simulink model "abl_M4_rigidPPC"  (R2023b)
settings: Solver=ode45  StartTime=0.0  StopTime=80  MaxStep=1e-3  RelTol=5e-5
model workspace (MAT data in the model file):
  gpsid1 : Simulink.Signal (value not decoded)
  gpsid2 : Simulink.Signal (value not decoded)
  gpsid3 : Simulink.Signal (value not decoded)
  kkk1 : Simulink.Signal (value not decoded)
  kkk2 : Simulink.Signal (value not decoded)
  kkk3 : Simulink.Signal (value not decoded)
  psid = 0.5
undefined symbols (not defined in the file): A_raw1, A_raw2, beta1, beta2, p00, p_d_10, p_d_20, p_d_30, p_d_40, p_d_50, p_d_60, p_hat_p10, p_hat_p20, p_hat_p30, p_hat_p40, p_hat_p50, p_hat_p60, p_hat_v10, p_hat_v20, p_hat_v30, p_hat_v40, p_hat_v50, p_hat_v60, p_off_set1, p_off_set2, v00
(part 3 of 4)

== matlab function abl_M4_rigidPPC/Subsystem12/Controler1 ==
  settings: updateMethod=DISCRETE
  data: t input; psi_d input; dpsid input; ddpsid input; psi_e input; rho_e input; tau_sat_rho output; tau_sat_psi output; alpha_psi output; alpha_rho output; B_psi output; B_rho output; z_rho output; desire input; u input; v input; r input; mu_rho_hat input; mu_psi_hat input; kappa_rho input; kappa_psi input; dot_mu_rho_hat output; dot_mu_psi_hat output; d_kappa_rho output; d_kappa_psi output; d_chi_rho_1 output; d_chi_rho_2 output; d_chi_psi_1 output; d_chi_psi_2 output; chi_rho_1 input; chi_rho_2 input; chi_psi_1 input; chi_psi_2 input; S_rho input; S_psi input; d_S_rho output; d_S_psi output
% function [tau_u,tau_r,alpha_psi,alpha_rho,dot_mu_rho_hat,dot_mu_psi_hat,sigma_rho,sigma_psi,z_rho,z_psi,term1 ,dpsie] = controller(t,psi_d,dpsid,ddpsid,psi_e, rho_e,desire,u, v, r,mu_rho_hat,mu_psi_hat)
% dxd = desire(2);ddxd = desire(3);dyd = desire(5);ddyd = desire(6);
% dpsie = r-dpsid;
% drhoe = u*cos(psi_e)+v*sin(psi_e)-dxd*cos(psi_d)-dyd*sin(psi_d);

% % epsilon = 0.05;

% % varkappa_rho =0.001;varkappa_psi=0.0005;
% % varpi_rho =2;varpi_psi =10;
% % k_rho=1.5;k_psi=10;
% % if rho_e<0.07
% %    varpi_rho =20;
% % end
% % if psi_e<0.1
% %    varpi_psi =50;
% % end
% % Tc_rho =16;Tc_psi =5;alpha=0.8;
% % sigma_rho0 =5;sigma_psi0 =2;
% % sigma_rho_inf =0.2;sigma_psi_inf=0.05;
% % Phi_rho=6*7;Phi_psi=8*7;
% 
% m11=25.8;m33=2.76;
% epsilon = 0.05;

% varkappa_rho =0.01;varkappa_psi=0.08;
% varpi_rho =1;varpi_psi =0.001;
% k_rho=100;k_psi=10;
% % if rho_e<0.07
% %    varpi_rho =20;
% % end
% % if psi_e<0.1
% %    varpi_psi =50;
% % end
% Tc_rho =25;Tc_psi =6;alpha=0.8;
% sigma_rho0 =20;sigma_psi0 =3;
% sigma_rho_inf =0.5;sigma_psi_inf=0.2;
% Phi_rho=0.01;Phi_psi=1;
% 

% 
% if t < Tc_rho
%      q_rho = 1-sin(pi*t/(2*Tc_rho));
%      dq_rho = -cos(pi*t/(2*Tc_rho))*pi/(2*Tc_rho);
% else
%     q_rho=0;
%     dq_rho=0;
% end
% if t < Tc_psi
%      q_psi = 1-sin(pi*t/(2*Tc_psi));
%      dq_psi = -cos(pi*t/(2*Tc_psi))*pi/(2*Tc_psi);
% else
%     q_psi = 0;
%     dq_psi=0;
% end
% 
% sigma_rho = (sigma_rho0 - sigma_rho_inf) * q_rho + sigma_rho_inf;
% sigma_psi = (sigma_psi0 - sigma_psi_inf) * q_psi + sigma_psi_inf;
% dsigma_rho = (sigma_rho0 - sigma_rho_inf)*dq_rho;
% dsigma_psi = (sigma_psi0 - sigma_psi_inf)*dq_psi;
% 
% alpha_rho =(1/sigma_rho^2)*(rho_e*sigma_rho*dsigma_rho-0.5*k_rho*(sigma_rho^2-rho_e^2)*rho_e-0*rho_e);
% alpha_psi =(1/sigma_psi^2)*(psi_e*sigma_psi*dsigma_psi-0.5*k_psi*(sigma_psi^2-psi_e^2)*psi_e);




function [tau_sat_rho,tau_sat_psi,alpha_psi, alpha_rho,B_psi,B_rho, z_rho, dot_mu_rho_hat, dot_mu_psi_hat, d_kappa_rho, d_kappa_psi,d_chi_rho_1,d_chi_rho_2,d_chi_psi_1,d_chi_psi_2,d_S_rho,d_S_psi] = LowLevel_Controller(t, psi_d,dpsid,ddpsid,psi_e, rho_e,desire,u, v, r,mu_rho_hat,mu_psi_hat,kappa_rho, kappa_psi,chi_rho_1,chi_rho_2,chi_psi_1,chi_psi_2,S_rho,S_psi)
    dxd = desire(2);ddxd = desire(3);dyd = desire(5);ddyd = desire(6);
    d_psi_e = r-dpsid;
    d_rho_e = u*cos(psi_e)-v*sin(psi_e)-dxd*cos(psi_d)-dyd*sin(psi_d); 
   % 移动目标围捕底层控制：预设时间与预设精度障碍李雅普诺夫控制器
    %
    % id: 当前智能体编号
    % A_raw: 全局通信拓扑矩阵 (NxN)
    
   %% ================= 0. 拓扑切换自动重启与初值捕获机制 =================
    persistent rho_e_0 psi_e_0;
    
    % 初始化阶段 (t = 0)
    if isempty(rho_e_0)
        rho_e_0 = rho_e;
        psi_e_0 = psi_e;
    end
   
    
    % Tracking PPC keeps the original time base; topology restart is handled in observer/guidance.
    t_local = t;

    %% ================= 1. 控制器参数配置 =================
    %Tc = 10.0; % 预设收敛时间 T_c
    
    % --- 径向误差(rho)参数 ---
    upsilon_rho_0 = 10;     
    upsilon_rho_inf = 0.2;          
    omega_rho_1 = 5.5; omega_rho_2 = 5.5;       
    gamma1_rho = 0.35;        
    k_rho_1 = 1.0;           
    k_rho_2 = 1.0;              
    Phi_rho=1;Phi_psi=2;
    K_psi = 135;K_rho = 0.018;
    m11=24.9;m33=2.86;
    h= 1/m33;
    g = cos(psi_e)/m11;

    % --- 航向误差(psi)参数 ---
    upsilon_psi_0 = 2*pi/5; 
    upsilon_psi_inf = 0.02;
    omega_psi_1 = 1; omega_psi_2 = 1;
    gamma1_psi = 4.0;
    k_psi_1 = 1.0;
    k_psi_2 = 1.0;  
    epsilon = 0.03;

    a_rho_1 = 300;a_rho_2 = 1000;b_rho_1 = 1;b_rho_2 = 1;
    a_psi_1 = 1000;a_psi_2 = 1000;b_psi_1 = 1;b_psi_2 = 1;
    wp_rho =0.001;wp_psi=0.001;
    varphi_rho =2;varphi_psi =1;
    %% ================= 2. 预设时间收敛函数 (使用 t_local 重启) =================
    % 严格对应公式 (0.4)
    Tc_psi = 2;
    if t_local < Tc_psi
        iota_psi = 1 - sin(pi * t_local / (2 * Tc_psi));
        d_iota_psi = -(pi / (2 * Tc_psi)) * cos(pi * t_local / (2 * Tc_psi));
    else
        iota_psi = 0;
        d_iota_psi = 0;
    end

    Tc_rho = 10;
    if t_local < Tc_rho
        iota_rho = 1 - sin(pi * t_local / (2 * Tc_rho));
        d_iota_rho = -(pi / (2 * Tc_rho)) * cos(pi * t_local / (2 * Tc_rho));
    else
        iota_rho = 0;
        d_iota_rho = 0;
    end

    %% ================= 3. 计算 rho 维度的控制量 =================
    N_rho = 1; if rho_e_0 < 0, N_rho = -1; end
    V_rho_0 = [1- N_rho; 1+N_rho];
    M_rho = [-1, -0.2; 0.2, 1];
    
    ups_rho = (upsilon_rho_0 - upsilon_rho_inf) * iota_rho + upsilon_rho_inf;
    d_ups_rho = (upsilon_rho_0 - upsilon_rho_inf) * d_iota_rho;
    
    b_rho = 0.5 * ups_rho * M_rho * V_rho_0 + rho_e_0 * iota_rho * [1; 1];
    d_b_rho = 0.5 * d_ups_rho * M_rho * V_rho_0 + rho_e_0 * d_iota_rho * [1; 1];
    d_kappa_rho = -k_rho_1 * kappa_rho + k_rho_2 * (chi_rho_1 + chi_rho_2);
    
    Omega_rho = [-omega_rho_1; omega_rho_2];
    B_rho = b_rho; % Ablation M4: rigid PPC, no elastic relaxation
    d_B_rho = d_b_rho;
    
    B_rho_lower = B_rho(1); B_rho_upper = B_rho(2);
    d_B_rho_lower = d_B_rho(1); d_B_rho_upper = d_B_rho(2);
    
    xi_rho = rho_e;
    B_diff_rho = B_rho_upper - B_rho_lower;
    
    theta_rho = (xi_rho - B_rho_lower) / B_diff_rho;
    
    phi_tan_rho = tan(pi * (theta_rho - 0.5));
    
    varpi_rho = (2 * pi * sec(pi * (theta_rho - 0.5))^2) / B_diff_rho;
    mu_rho = varpi_rho * (-rho_e_0 * d_iota_rho - d_B_rho_lower - ...
             (xi_rho - B_rho_lower) / B_diff_rho * (d_B_rho_upper - d_B_rho_lower));
             
    alpha_rho = (1 / varpi_rho) * (-sign(varpi_rho)*varpi_rho*gamma1_rho * phi_tan_rho - mu_rho) - S_rho;
    z_rho = d_rho_e - alpha_rho - S_rho; 

    %% ================= 4. 计算 psi 维度的控制量 =================
    N_psi = 1; if psi_e_0 < 0, N_psi = -1; end
    V_psi_0 = [1-N_psi; 1+N_psi];
    M_psi = [-1, 0.2; 0.2, 1];
    
    ups_psi = (upsilon_psi_0 - upsilon_psi_inf) * iota_psi + upsilon_psi_inf;
    d_ups_psi = (upsilon_psi_0 - upsilon_psi_inf) * d_iota_psi;
    
    b_psi = 0.5 * ups_psi * M_psi * V_psi_0 + psi_e_0 * iota_psi * [1; 1];
    d_b_psi = 0.5 * d_ups_psi * M_psi * V_psi_0 + psi_e_0 * d_iota_psi * [1; 1];
    d_kappa_psi = -k_psi_1 * kappa_psi + k_psi_2 * (chi_psi_1 + chi_psi_2);
    
    Omega_psi = [-omega_psi_1; omega_psi_2];
    B_psi = b_psi; % Ablation M4: rigid PPC, no elastic relaxation
    d_B_psi = d_b_psi;
    
    B_psi_lower = B_psi(1); B_psi_upper = B_psi(2);
    d_B_psi_lower = d_B_psi(1); d_B_psi_upper = d_B_psi(2);
    
    xi_psi = psi_e;
    B_diff_psi = B_psi_upper - B_psi_lower;
    theta_psi = (xi_psi - B_psi_lower) / B_diff_psi;
    
    
    phi_tan_psi = tan(pi * (theta_psi - 0.5));
    
    varpi_psi = (2 * pi * sec(pi * (theta_psi - 0.5))^2) / B_diff_psi;
    mu_psi = varpi_psi * (-psi_e_0 * d_iota_psi - d_B_psi_lower - ...
             (xi_psi - B_psi_lower) / B_diff_psi * (d_B_psi_upper - d_B_psi_lower));
             
    alpha_psi = (1 / varpi_psi) * (-sign(varpi_psi)*varpi_psi*gamma1_psi * phi_tan_psi - mu_psi) - S_psi;
    z_psi = d_psi_e - alpha_psi - S_psi; 
    
    % kappa_rho = 2*rho_e*sigma_rho^2/(sigma_rho^2 - rho_e^2)^2;
    % kappa_psi = 2*psi_e*sigma_psi^2/(sigma_psi^2 - psi_e^2)^2;
    
    vartheta_rho = norm(NN([alpha_rho,rho_e])) + 1;
    vartheta_psi = norm(NN([alpha_psi,psi_e])) + 1;
    
    term1=tanh(mu_rho_hat *Phi_rho^2* z_rho^2 * vartheta_rho^2 / epsilon);
    term2=tanh(mu_psi_hat *Phi_psi^2* z_psi^2 * vartheta_psi^2 / epsilon);
    
    tau_u = -(1/g) * (0.5 * K_rho * z_rho + 0.5*mu_rho_hat * vartheta_rho^2 *Phi_rho^2* z_rho * term1);
    tau_r = -(1/h) * (0.5 * K_psi * z_psi + 0.5*mu_psi_hat * vartheta_psi^2 *Phi_psi^2* z_psi * term2);
    
    dot_mu_rho_hat = -wp_rho * (-0.5 * vartheta_rho^2*Phi_rho^2*z_rho^2 + varphi_rho * mu_rho_hat);
    dot_mu_psi_hat = -wp_psi * (-0.5 * vartheta_psi^2*Phi_psi^2*z_psi^2 + varphi_psi * mu_psi_hat);
    

    tau_bu_psi = 400;tau_bu_rho = 800;
    term_rho_1 = (sign(tau_u - tau_bu_rho) + 1) * (tau_u - tau_bu_rho);
    term_rho_2 = (sign(tau_u + tau_bu_rho) - 1) * (tau_u + tau_bu_rho);
    d_chi_rho_1 = -a_rho_1 * chi_rho_1 + b_rho_1 * term_rho_1;
    d_chi_rho_2 = -a_rho_2 * chi_rho_2 + b_rho_2 * term_rho_2;
    term_psi_1 = (sign(tau_r - tau_bu_psi) + 1) * (tau_r - tau_bu_psi);
    term_psi_2 = (sign(tau_r + tau_bu_psi) - 1) * (tau_r + tau_bu_psi);
    d_chi_psi_1 = -a_psi_1 * chi_psi_1 + b_psi_1 * term_psi_1;
    d_chi_psi_2 = -a_psi_2 * chi_psi_2 + b_psi_2 * term_psi_2;
    % 模拟实际限幅函数 g(tau)
    G_psi = h;G_rho = g;
    tau_sat_psi = max(min(tau_r, tau_bu_psi), -tau_bu_psi);
    d_S_psi = -S_psi + G_psi * (tau_sat_psi - tau_r);
    % 模拟实际限幅函数 g(tau)
    tau_sat_rho = max(min(tau_u, tau_bu_rho), -tau_bu_rho); 
    d_S_rho = -S_rho + G_rho * (tau_sat_rho - tau_u);
end

 function NNv= NN(theta)
    NNv = zeros(50,1);
    for i=1:50
        paran = 0.005*i;
        param = ones(length(theta),1)*sin(0.1*i);
        NNv(i) = exp(-norm(theta-param)^2/paran);
    end
end

== matlab function abl_M4_rigidPPC/Subsystem12/Subsystem/Guidence ==
  settings: updateMethod=DISCRETE
  data: t input; x input; y input; desire input; psi input; psid output; psi_e output; rhoe output; xd output; yd output
function [psid,psi_e,rhoe,xd,yd]  = desire(t,x,y,desire,psi)
xd = desire(1);yd = desire(4);
dxd = desire(2); dyd=desire(5);
xe =x-xd;
ye =y-yd;
 rhoe = sqrt((xe)^2+(ye)^2); 
 persistent kkk4 gpsid4
% if abs(rhoe)<1
    p = atan2(10000*ye+10*dyd,10000*xe+10*dxd);
    % u1 = 0.1*dxd+10*xe;
    % u2 = 0.1*dyd+10*ye;
    % z=u1+u2*i;
    % p=angle(z);
% else
%     p = atan2(ye,xe);
% end

if isempty(kkk4)
    kkk4=0;
    gpsid4=p;
end
if p*gpsid4<-0.7*pi^2 && p>0  %Change nearly in -pi and +pi
   kkk4=kkk4-1;
end
if p*gpsid4<-0.7*pi^2 && p<0  %Change nearly in -pi and +pi
   kkk4=kkk4+1;
end
gpsid4=p;
psid=p+2*kkk4*pi;
psi_e = psi-psid;
 
 

end

== matlab function abl_M4_rigidPPC/Subsystem12/Subsystem1/MATLAB Function1 ==
  data: x1 input; dotx1 output; dotx2 output; x2 input; psid input
function [dotx1,dotx2] = desire(x1,x2,psid)
    R  = 1;
    dotx1 = x2;
    dotx2 = -2*R^2*(x1-psid)-R*x2;
end

== matlab function abl_M4_rigidPPC/Subsystem12/Subsystem1/MATLAB Function2 ==
  data: x1 input; dotx1 output; dotx2 output; x2 input; psid input
function [dotx1,dotx2] = desire(x1,x2,psid)
    R  = 1;
    dotx1 = x2;
    dotx2 = -2*R^2*(x1-psid)-R*x2;
end

== matlab function abl_M4_rigidPPC/USV3/MATLAB Function ==
  data: t input; tau_u input; x_dot output; y_dot output; psi_dot output; u_dot output; v_dot output; r_dot output; tau_r input; psi input; u input; v input; r input
function [x_dot, y_dot, psi_dot, u_dot, v_dot, r_dot] = dynamics(t,tau_u,tau_r,psi,u, v, r)
    m11=24.9;m22=33.8;m33=2.86;
    Du=12;Dv=17;Dr=0.5;
    % Kinematic equations
    x_dot = u * cos(psi) - v * sin(psi);
    y_dot = u * sin(psi) + v * cos(psi);    
    psi_dot = r;
    % Disturbence
    tau_wu = 0.50*sin(0.1*t);
    tau_wv = 0.50*cos(0.1*t); 
    tau_wr = 0.50*sin(0.2*t);
    % Dynamic equations
    u_dot = (m22 * v * r - Du * u + tau_u + tau_wu) / m11;
    v_dot = (-m11 * u * r - Dv * v + tau_wv) / m22;
    r_dot = ((m11 - m22) * u * v - Dr * r + tau_r + tau_wr) / m33;
    % 质量和惯性参数
   

end

== matlab function abl_M4_rigidPPC/Subsystem13/MATLAB Function8 ==
  data: x1 input; dotx1 output; dotx2 output; x2 input; dpd input
function [dotx1,dotx2] = desire(x1,x2,dpd)
    R  = 1;
    dotx1 = x2;
    dotx2 = -2*R^2*(x1-dpd)-R*x2;
end

== matlab function abl_M4_rigidPPC/Subsystem13/MATLAB Function9 ==
  data: x1 input; dotx1 output; dotx2 output; x2 input; pd input
function [dotx1,dotx2] = desire(x1,x2,pd)
    R  = 5;
    dotx1 = x2;
    dotx2 = -2*R^2*(x1-pd)-R*x2;
end

== matlab function abl_M4_rigidPPC/Subsystem14/Controler1 ==
  settings: updateMethod=DISCRETE
  data: t input; psi_d input; dpsid input; ddpsid input; psi_e input; rho_e input; tau_sat_rho output; tau_sat_psi output; alpha_psi output; alpha_rho output; B_psi output; B_rho output; z_rho output; desire input; u input; v input; r input; mu_rho_hat input; mu_psi_hat input; kappa_rho input; kappa_psi input; dot_mu_rho_hat output; dot_mu_psi_hat output; d_kappa_rho output; d_kappa_psi output; d_chi_rho_1 output; d_chi_rho_2 output; d_chi_psi_1 output; d_chi_psi_2 output; chi_rho_1 input; chi_rho_2 input; chi_psi_1 input; chi_psi_2 input; S_rho input; S_psi input; d_S_rho output; d_S_psi output
% function [tau_u,tau_r,alpha_psi,alpha_rho,dot_mu_rho_hat,dot_mu_psi_hat,sigma_rho,sigma_psi,z_rho,z_psi,term1 ,dpsie] = controller(t,psi_d,dpsid,ddpsid,psi_e, rho_e,desire,u, v, r,mu_rho_hat,mu_psi_hat)
% dxd = desire(2);ddxd = desire(3);dyd = desire(5);ddyd = desire(6);
% dpsie = r-dpsid;
% drhoe = u*cos(psi_e)+v*sin(psi_e)-dxd*cos(psi_d)-dyd*sin(psi_d);

% % epsilon = 0.05;

% % varkappa_rho =0.001;varkappa_psi=0.0005;
% % varpi_rho =2;varpi_psi =10;
% % k_rho=1.5;k_psi=10;
% % if rho_e<0.07
% %    varpi_rho =20;
% % end
% % if psi_e<0.1
% %    varpi_psi =50;
% % end
% % Tc_rho =16;Tc_psi =5;alpha=0.8;
% % sigma_rho0 =5;sigma_psi0 =2;
% % sigma_rho_inf =0.2;sigma_psi_inf=0.05;
% % Phi_rho=6*7;Phi_psi=8*7;
% 
% m11=25.8;m33=2.76;
% epsilon = 0.05;

% varkappa_rho =0.01;varkappa_psi=0.08;
% varpi_rho =1;varpi_psi =0.001;
% k_rho=100;k_psi=10;
% % if rho_e<0.07
% %    varpi_rho =20;
% % end
% % if psi_e<0.1
% %    varpi_psi =50;
% % end
% Tc_rho =25;Tc_psi =6;alpha=0.8;
% sigma_rho0 =20;sigma_psi0 =3;
% sigma_rho_inf =0.5;sigma_psi_inf=0.2;
% Phi_rho=0.01;Phi_psi=1;
% 

% 
% if t < Tc_rho
%      q_rho = 1-sin(pi*t/(2*Tc_rho));
%      dq_rho = -cos(pi*t/(2*Tc_rho))*pi/(2*Tc_rho);
% else
%     q_rho=0;
%     dq_rho=0;
% end
% if t < Tc_psi
%      q_psi = 1-sin(pi*t/(2*Tc_psi));
%      dq_psi = -cos(pi*t/(2*Tc_psi))*pi/(2*Tc_psi);
% else
%     q_psi = 0;
%     dq_psi=0;
% end
% 
% sigma_rho = (sigma_rho0 - sigma_rho_inf) * q_rho + sigma_rho_inf;
% sigma_psi = (sigma_psi0 - sigma_psi_inf) * q_psi + sigma_psi_inf;
% dsigma_rho = (sigma_rho0 - sigma_rho_inf)*dq_rho;
% dsigma_psi = (sigma_psi0 - sigma_psi_inf)*dq_psi;
% 
% alpha_rho =(1/sigma_rho^2)*(rho_e*sigma_rho*dsigma_rho-0.5*k_rho*(sigma_rho^2-rho_e^2)*rho_e-0*rho_e);
% alpha_psi =(1/sigma_psi^2)*(psi_e*sigma_psi*dsigma_psi-0.5*k_psi*(sigma_psi^2-psi_e^2)*psi_e);




function [tau_sat_rho,tau_sat_psi,alpha_psi, alpha_rho,B_psi,B_rho, z_rho, dot_mu_rho_hat, dot_mu_psi_hat, d_kappa_rho, d_kappa_psi,d_chi_rho_1,d_chi_rho_2,d_chi_psi_1,d_chi_psi_2,d_S_rho,d_S_psi] = LowLevel_Controller(t, psi_d,dpsid,ddpsid,psi_e, rho_e,desire,u, v, r,mu_rho_hat,mu_psi_hat,kappa_rho, kappa_psi,chi_rho_1,chi_rho_2,chi_psi_1,chi_psi_2,S_rho,S_psi)
    dxd = desire(2);ddxd = desire(3);dyd = desire(5);ddyd = desire(6);
    d_psi_e = r-dpsid;
    d_rho_e = u*cos(psi_e)-v*sin(psi_e)-dxd*cos(psi_d)-dyd*sin(psi_d); 
   % 移动目标围捕底层控制：预设时间与预设精度障碍李雅普诺夫控制器
    %
    % id: 当前智能体编号
    % A_raw: 全局通信拓扑矩阵 (NxN)
    
   %% ================= 0. 拓扑切换自动重启与初值捕获机制 =================
    persistent rho_e_0 psi_e_0;
    
    % 初始化阶段 (t = 0)
    if isempty(rho_e_0)
        rho_e_0 = rho_e;
        psi_e_0 = psi_e;
    end
   
    
    % Tracking PPC keeps the original time base; topology restart is handled in observer/guidance.
    t_local = t;

    %% ================= 1. 控制器参数配置 =================
    %Tc = 10.0; % 预设收敛时间 T_c
    
    % --- 径向误差(rho)参数 ---
    upsilon_rho_0 = 10;     
    upsilon_rho_inf = 0.2;          
    omega_rho_1 = 5.5; omega_rho_2 = 5.5;       
    gamma1_rho = 0.35;        
    k_rho_1 = 1.0;           
    k_rho_2 = 1.0;              
    Phi_rho=1;Phi_psi=2;
    K_psi = 135;K_rho = 0.018;
    m11=24.9;m33=2.86;
    h= 1/m33;
    g = cos(psi_e)/m11;

    % --- 航向误差(psi)参数 ---
    upsilon_psi_0 = 2*pi/5; 
    upsilon_psi_inf = 0.02;
    omega_psi_1 = 1; omega_psi_2 = 1;
    gamma1_psi = 4.0;
    k_psi_1 = 1.0;
    k_psi_2 = 1.0;  
    epsilon = 0.03;

    a_rho_1 = 300;a_rho_2 = 1000;b_rho_1 = 1;b_rho_2 = 1;
    a_psi_1 = 1000;a_psi_2 = 1000;b_psi_1 = 1;b_psi_2 = 1;
    wp_rho =0.001;wp_psi=0.001;
    varphi_rho =2;varphi_psi =1;
    %% ================= 2. 预设时间收敛函数 (使用 t_local 重启) =================
    % 严格对应公式 (0.4)
    Tc_psi = 2;
    if t_local < Tc_psi
        iota_psi = 1 - sin(pi * t_local / (2 * Tc_psi));
        d_iota_psi = -(pi / (2 * Tc_psi)) * cos(pi * t_local / (2 * Tc_psi));
    else
        iota_psi = 0;
        d_iota_psi = 0;
    end

    Tc_rho = 10;
    if t_local < Tc_rho
        iota_rho = 1 - sin(pi * t_local / (2 * Tc_rho));
        d_iota_rho = -(pi / (2 * Tc_rho)) * cos(pi * t_local / (2 * Tc_rho));
    else
        iota_rho = 0;
        d_iota_rho = 0;
    end

    %% ================= 3. 计算 rho 维度的控制量 =================
    N_rho = 1; if rho_e_0 < 0, N_rho = -1; end
    V_rho_0 = [1- N_rho; 1+N_rho];
    M_rho = [-1, -0.2; 0.2, 1];
    
    ups_rho = (upsilon_rho_0 - upsilon_rho_inf) * iota_rho + upsilon_rho_inf;
    d_ups_rho = (upsilon_rho_0 - upsilon_rho_inf) * d_iota_rho;
    
    b_rho = 0.5 * ups_rho * M_rho * V_rho_0 + rho_e_0 * iota_rho * [1; 1];
    d_b_rho = 0.5 * d_ups_rho * M_rho * V_rho_0 + rho_e_0 * d_iota_rho * [1; 1];
    d_kappa_rho = -k_rho_1 * kappa_rho + k_rho_2 * (chi_rho_1 + chi_rho_2);
    
    Omega_rho = [-omega_rho_1; omega_rho_2];
    B_rho = b_rho; % Ablation M4: rigid PPC, no elastic relaxation
    d_B_rho = d_b_rho;
    
    B_rho_lower = B_rho(1); B_rho_upper = B_rho(2);
    d_B_rho_lower = d_B_rho(1); d_B_rho_upper = d_B_rho(2);
    
    xi_rho = rho_e;
    B_diff_rho = B_rho_upper - B_rho_lower;
    
    theta_rho = (xi_rho - B_rho_lower) / B_diff_rho;
    
    phi_tan_rho = tan(pi * (theta_rho - 0.5));
    
    varpi_rho = (2 * pi * sec(pi * (theta_rho - 0.5))^2) / B_diff_rho;
    mu_rho = varpi_rho * (-rho_e_0 * d_iota_rho - d_B_rho_lower - ...
             (xi_rho - B_rho_lower) / B_diff_rho * (d_B_rho_upper - d_B_rho_lower));
             
    alpha_rho = (1 / varpi_rho) * (-sign(varpi_rho)*varpi_rho*gamma1_rho * phi_tan_rho - mu_rho) - S_rho;
    z_rho = d_rho_e - alpha_rho - S_rho; 

    %% ================= 4. 计算 psi 维度的控制量 =================
    N_psi = 1; if psi_e_0 < 0, N_psi = -1; end
    V_psi_0 = [1-N_psi; 1+N_psi];
    M_psi = [-1, 0.2; 0.2, 1];
    
    ups_psi = (upsilon_psi_0 - upsilon_psi_inf) * iota_psi + upsilon_psi_inf;
    d_ups_psi = (upsilon_psi_0 - upsilon_psi_inf) * d_iota_psi;
    
    b_psi = 0.5 * ups_psi * M_psi * V_psi_0 + psi_e_0 * iota_psi * [1; 1];
    d_b_psi = 0.5 * d_ups_psi * M_psi * V_psi_0 + psi_e_0 * d_iota_psi * [1; 1];
    d_kappa_psi = -k_psi_1 * kappa_psi + k_psi_2 * (chi_psi_1 + chi_psi_2);
    
    Omega_psi = [-omega_psi_1; omega_psi_2];
    B_psi = b_psi; % Ablation M4: rigid PPC, no elastic relaxation
    d_B_psi = d_b_psi;
    
    B_psi_lower = B_psi(1); B_psi_upper = B_psi(2);
    d_B_psi_lower = d_B_psi(1); d_B_psi_upper = d_B_psi(2);
    
    xi_psi = psi_e;
    B_diff_psi = B_psi_upper - B_psi_lower;
    theta_psi = (xi_psi - B_psi_lower) / B_diff_psi;
    
    
    phi_tan_psi = tan(pi * (theta_psi - 0.5));
    
    varpi_psi = (2 * pi * sec(pi * (theta_psi - 0.5))^2) / B_diff_psi;
    mu_psi = varpi_psi * (-psi_e_0 * d_iota_psi - d_B_psi_lower - ...
             (xi_psi - B_psi_lower) / B_diff_psi * (d_B_psi_upper - d_B_psi_lower));
             
    alpha_psi = (1 / varpi_psi) * (-sign(varpi_psi)*varpi_psi*gamma1_psi * phi_tan_psi - mu_psi) - S_psi;
    z_psi = d_psi_e - alpha_psi - S_psi; 
    
    % kappa_rho = 2*rho_e*sigma_rho^2/(sigma_rho^2 - rho_e^2)^2;
    % kappa_psi = 2*psi_e*sigma_psi^2/(sigma_psi^2 - psi_e^2)^2;
    
    vartheta_rho = norm(NN([alpha_rho,rho_e])) + 1;
    vartheta_psi = norm(NN([alpha_psi,psi_e])) + 1;
    
    term1=tanh(mu_rho_hat *Phi_rho^2* z_rho^2 * vartheta_rho^2 / epsilon);
    term2=tanh(mu_psi_hat *Phi_psi^2* z_psi^2 * vartheta_psi^2 / epsilon);
    
    tau_u = -(1/g) * (0.5 * K_rho * z_rho + 0.5*mu_rho_hat * vartheta_rho^2 *Phi_rho^2* z_rho * term1);
    tau_r = -(1/h) * (0.5 * K_psi * z_psi + 0.5*mu_psi_hat * vartheta_psi^2 *Phi_psi^2* z_psi * term2);
    
    dot_mu_rho_hat = -wp_rho * (-0.5 * vartheta_rho^2*Phi_rho^2*z_rho^2 + varphi_rho * mu_rho_hat);
    dot_mu_psi_hat = -wp_psi * (-0.5 * vartheta_psi^2*Phi_psi^2*z_psi^2 + varphi_psi * mu_psi_hat);
    

    tau_bu_psi = 400;tau_bu_rho = 800;
    term_rho_1 = (sign(tau_u - tau_bu_rho) + 1) * (tau_u - tau_bu_rho);
    term_rho_2 = (sign(tau_u + tau_bu_rho) - 1) * (tau_u + tau_bu_rho);
    d_chi_rho_1 = -a_rho_1 * chi_rho_1 + b_rho_1 * term_rho_1;
    d_chi_rho_2 = -a_rho_2 * chi_rho_2 + b_rho_2 * term_rho_2;
    term_psi_1 = (sign(tau_r - tau_bu_psi) + 1) * (tau_r - tau_bu_psi);
    term_psi_2 = (sign(tau_r + tau_bu_psi) - 1) * (tau_r + tau_bu_psi);
    d_chi_psi_1 = -a_psi_1 * chi_psi_1 + b_psi_1 * term_psi_1;
    d_chi_psi_2 = -a_psi_2 * chi_psi_2 + b_psi_2 * term_psi_2;
    % 模拟实际限幅函数 g(tau)
    G_psi = h;G_rho = g;
    tau_sat_psi = max(min(tau_r, tau_bu_psi), -tau_bu_psi);
    d_S_psi = -S_psi + G_psi * (tau_sat_psi - tau_r);
    % 模拟实际限幅函数 g(tau)
    tau_sat_rho = max(min(tau_u, tau_bu_rho), -tau_bu_rho); 
    d_S_rho = -S_rho + G_rho * (tau_sat_rho - tau_u);
end

 function NNv= NN(theta)
    NNv = zeros(50,1);
    for i=1:50
        paran = 0.005*i;
        param = ones(length(theta),1)*sin(0.1*i);
        NNv(i) = exp(-norm(theta-param)^2/paran);
    end
end

== matlab function abl_M4_rigidPPC/Subsystem14/Subsystem/Guidence ==
  settings: updateMethod=DISCRETE
  data: t input; x input; y input; desire input; psi input; psid output; psi_e output; rhoe output; xd output; yd output
function [psid,psi_e,rhoe,xd,yd]  = desire(t,x,y,desire,psi)
xd = desire(1);yd = desire(4);
dxd = desire(2); dyd=desire(5);
xe =x-xd;
ye =y-yd;
 rhoe = sqrt((xe)^2+(ye)^2); 
 persistent kkk2 gpsid2
% if abs(rhoe)<1
    p = atan2(10000*ye+10*dyd,10000*xe+10*dxd);
    % u1 = 0.1*dxd+10*xe;
    % u2 = 0.1*dyd+10*ye;
    % z=u1+u2*i;
    % p=angle(z);
% else
%     p = atan2(ye,xe);
% end

if isempty(kkk2)
    kkk2=0;
    gpsid2=p;
end
if p*gpsid2<-0.7*pi^2 && p>0  %Change nearly in -pi and +pi
   kkk2=kkk2-1;
end
if p*gpsid2<-0.7*pi^2 && p<0  %Change nearly in -pi and +pi
   kkk2=kkk2+1;
end
gpsid2=p;
psid=p+2*kkk2*pi;
psi_e = psi-psid;
 
 

end

== matlab function abl_M4_rigidPPC/Subsystem14/Subsystem1/MATLAB Function1 ==
  data: x1 input; dotx1 output; dotx2 output; x2 input; psid input
function [dotx1,dotx2] = desire(x1,x2,psid)
    R  = 1;
    dotx1 = x2;
    dotx2 = -2*R^2*(x1-psid)-R*x2;
end

== matlab function abl_M4_rigidPPC/Subsystem14/Subsystem1/MATLAB Function2 ==
  data: x1 input; dotx1 output; dotx2 output; x2 input; psid input
function [dotx1,dotx2] = desire(x1,x2,psid)
    R  = 1;
    dotx1 = x2;
    dotx2 = -2*R^2*(x1-psid)-R*x2;
end

== matlab function abl_M4_rigidPPC/USV7/MATLAB Function ==
  data: t input; tau_u input; x_dot output; y_dot output; psi_dot output; u_dot output; v_dot output; r_dot output; tau_r input; psi input; u input; v input; r input
function [x_dot, y_dot, psi_dot, u_dot, v_dot, r_dot] = dynamics(t,tau_u,tau_r,psi,u, v, r)
    m11=24.9;m22=33.8;m33=2.86;
    Du=12;Dv=17;Dr=0.5;
    % Kinematic equations
    x_dot = u * cos(psi) - v * sin(psi);
    y_dot = u * sin(psi) + v * cos(psi);    
    psi_dot = r;
    % Disturbence
    tau_wu = 0.50*sin(0.1*t);
    tau_wv = 0.50*cos(0.1*t); 
    tau_wr = 0.50*sin(0.2*t);
    % Dynamic equations
    u_dot = (m22 * v * r - Du * u + tau_u + tau_wu) / m11;
    v_dot = (-m11 * u * r - Dv * v + tau_wv) / m22;
    r_dot = ((m11 - m22) * u * v - Dr * r + tau_r + tau_wr) / m33;
    % 质量和惯性参数
   

end

== matlab function abl_M4_rigidPPC/Subsystem15/MATLAB Function8 ==
  data: x1 input; dotx1 output; dotx2 output; x2 input; dpd input
function [dotx1,dotx2] = desire(x1,x2,dpd)
    R  = 1;
    dotx1 = x2;
    dotx2 = -2*R^2*(x1-dpd)-R*x2;
end

== matlab function abl_M4_rigidPPC/Subsystem15/MATLAB Function9 ==
  data: x1 input; dotx1 output; dotx2 output; x2 input; pd input
function [dotx1,dotx2] = desire(x1,x2,pd)
    R  = 10;
    dotx1 = x2;
    dotx2 = -2*R^2*(x1-pd)-R*x2;
end

== matlab function abl_M4_rigidPPC/Subsystem16/Controler1 ==
  settings: updateMethod=DISCRETE
  data: t input; psi_d input; dpsid input; ddpsid input; psi_e input; rho_e input; tau_sat_rho output; tau_sat_psi output; alpha_psi output; alpha_rho output; B_psi output; B_rho output; z_rho output; desire input; u input; v input; r input; mu_rho_hat input; mu_psi_hat input; kappa_rho input; kappa_psi input; dot_mu_rho_hat output; dot_mu_psi_hat output; d_kappa_rho output; d_kappa_psi output; d_chi_rho_1 output; d_chi_rho_2 output; d_chi_psi_1 output; d_chi_psi_2 output; chi_rho_1 input; chi_rho_2 input; chi_psi_1 input; chi_psi_2 input; S_rho input; S_psi input; d_S_rho output; d_S_psi output
% function [tau_u,tau_r,alpha_psi,alpha_rho,dot_mu_rho_hat,dot_mu_psi_hat,sigma_rho,sigma_psi,z_rho,z_psi,term1 ,dpsie] = controller(t,psi_d,dpsid,ddpsid,psi_e, rho_e,desire,u, v, r,mu_rho_hat,mu_psi_hat)
% dxd = desire(2);ddxd = desire(3);dyd = desire(5);ddyd = desire(6);
% dpsie = r-dpsid;
% drhoe = u*cos(psi_e)+v*sin(psi_e)-dxd*cos(psi_d)-dyd*sin(psi_d);

% % epsilon = 0.05;

% % varkappa_rho =0.001;varkappa_psi=0.0005;
% % varpi_rho =2;varpi_psi =10;
% % k_rho=1.5;k_psi=10;
% % if rho_e<0.07
% %    varpi_rho =20;
% % end
% % if psi_e<0.1
% %    varpi_psi =50;
% % end
% % Tc_rho =16;Tc_psi =5;alpha=0.8;
% % sigma_rho0 =5;sigma_psi0 =2;
% % sigma_rho_inf =0.2;sigma_psi_inf=0.05;
% % Phi_rho=6*7;Phi_psi=8*7;
% 
% m11=25.8;m33=2.76;
% epsilon = 0.05;

% varkappa_rho =0.01;varkappa_psi=0.08;
% varpi_rho =1;varpi_psi =0.001;
% k_rho=100;k_psi=10;
% % if rho_e<0.07
% %    varpi_rho =20;
% % end
% % if psi_e<0.1
% %    varpi_psi =50;
% % end
% Tc_rho =25;Tc_psi =6;alpha=0.8;
% sigma_rho0 =20;sigma_psi0 =3;
% sigma_rho_inf =0.5;sigma_psi_inf=0.2;
% Phi_rho=0.01;Phi_psi=1;
% 

% 
% if t < Tc_rho
%      q_rho = 1-sin(pi*t/(2*Tc_rho));
%      dq_rho = -cos(pi*t/(2*Tc_rho))*pi/(2*Tc_rho);
% else
%     q_rho=0;
%     dq_rho=0;
% end
% if t < Tc_psi
%      q_psi = 1-sin(pi*t/(2*Tc_psi));
%      dq_psi = -cos(pi*t/(2*Tc_psi))*pi/(2*Tc_psi);
% else
%     q_psi = 0;
%     dq_psi=0;
% end
% 
% sigma_rho = (sigma_rho0 - sigma_rho_inf) * q_rho + sigma_rho_inf;
% sigma_psi = (sigma_psi0 - sigma_psi_inf) * q_psi + sigma_psi_inf;
% dsigma_rho = (sigma_rho0 - sigma_rho_inf)*dq_rho;
% dsigma_psi = (sigma_psi0 - sigma_psi_inf)*dq_psi;
% 
% alpha_rho =(1/sigma_rho^2)*(rho_e*sigma_rho*dsigma_rho-0.5*k_rho*(sigma_rho^2-rho_e^2)*rho_e-0*rho_e);
% alpha_psi =(1/sigma_psi^2)*(psi_e*sigma_psi*dsigma_psi-0.5*k_psi*(sigma_psi^2-psi_e^2)*psi_e);




function [tau_sat_rho,tau_sat_psi,alpha_psi, alpha_rho,B_psi,B_rho, z_rho, dot_mu_rho_hat, dot_mu_psi_hat, d_kappa_rho, d_kappa_psi,d_chi_rho_1,d_chi_rho_2,d_chi_psi_1,d_chi_psi_2,d_S_rho,d_S_psi] = LowLevel_Controller(t, psi_d,dpsid,ddpsid,psi_e, rho_e,desire,u, v, r,mu_rho_hat,mu_psi_hat,kappa_rho, kappa_psi,chi_rho_1,chi_rho_2,chi_psi_1,chi_psi_2,S_rho,S_psi)
    dxd = desire(2);ddxd = desire(3);dyd = desire(5);ddyd = desire(6);
    d_psi_e = r-dpsid;
    d_rho_e = u*cos(psi_e)-v*sin(psi_e)-dxd*cos(psi_d)-dyd*sin(psi_d); 
   % 移动目标围捕底层控制：预设时间与预设精度障碍李雅普诺夫控制器
    %
    % id: 当前智能体编号
    % A_raw: 全局通信拓扑矩阵 (NxN)
    
   %% ================= 0. 拓扑切换自动重启与初值捕获机制 =================
    persistent rho_e_0 psi_e_0;
    
    % 初始化阶段 (t = 0)
    if isempty(rho_e_0)
        rho_e_0 = rho_e;
        psi_e_0 = psi_e;
    end
   
    
    % Tracking PPC keeps the original time base; topology restart is handled in observer/guidance.
    t_local = t;

    %% ================= 1. 控制器参数配置 =================
    %Tc = 10.0; % 预设收敛时间 T_c
    
    % --- 径向误差(rho)参数 ---
    upsilon_rho_0 = 10;     
    upsilon_rho_inf = 0.2;          
    omega_rho_1 = 5.5; omega_rho_2 = 5.5;       
    gamma1_rho = 0.35;        
    k_rho_1 = 1.0;           
    k_rho_2 = 1.0;              
    Phi_rho=1;Phi_psi=2;
    K_psi = 135;K_rho = 0.018;
    m11=24.9;m33=2.86;
    h= 1/m33;
    g = cos(psi_e)/m11;

    % --- 航向误差(psi)参数 ---
    upsilon_psi_0 = 2*pi/5; 
    upsilon_psi_inf = 0.02;
    omega_psi_1 = 1; omega_psi_2 = 1;
    gamma1_psi = 4.0;
    k_psi_1 = 1.0;
    k_psi_2 = 1.0;  
    epsilon = 0.03;

    a_rho_1 = 300;a_rho_2 = 1000;b_rho_1 = 1;b_rho_2 = 1;
    a_psi_1 = 1000;a_psi_2 = 1000;b_psi_1 = 1;b_psi_2 = 1;
    wp_rho =0.001;wp_psi=0.001;
    varphi_rho =2;varphi_psi =1;
    %% ================= 2. 预设时间收敛函数 (使用 t_local 重启) =================
    % 严格对应公式 (0.4)
    Tc_psi = 2;
    if t_local < Tc_psi
        iota_psi = 1 - sin(pi * t_local / (2 * Tc_psi));
        d_iota_psi = -(pi / (2 * Tc_psi)) * cos(pi * t_local / (2 * Tc_psi));
    else
        iota_psi = 0;
        d_iota_psi = 0;
    end

    Tc_rho = 10;
    if t_local < Tc_rho
        iota_rho = 1 - sin(pi * t_local / (2 * Tc_rho));
        d_iota_rho = -(pi / (2 * Tc_rho)) * cos(pi * t_local / (2 * Tc_rho));
    else
        iota_rho = 0;
        d_iota_rho = 0;
    end

    %% ================= 3. 计算 rho 维度的控制量 =================
    N_rho = 1; if rho_e_0 < 0, N_rho = -1; end
    V_rho_0 = [1- N_rho; 1+N_rho];
    M_rho = [-1, -0.2; 0.2, 1];
    
    ups_rho = (upsilon_rho_0 - upsilon_rho_inf) * iota_rho + upsilon_rho_inf;
    d_ups_rho = (upsilon_rho_0 - upsilon_rho_inf) * d_iota_rho;
    
    b_rho = 0.5 * ups_rho * M_rho * V_rho_0 + rho_e_0 * iota_rho * [1; 1];
    d_b_rho = 0.5 * d_ups_rho * M_rho * V_rho_0 + rho_e_0 * d_iota_rho * [1; 1];
    d_kappa_rho = -k_rho_1 * kappa_rho + k_rho_2 * (chi_rho_1 + chi_rho_2);
    
    Omega_rho = [-omega_rho_1; omega_rho_2];
    B_rho = b_rho; % Ablation M4: rigid PPC, no elastic relaxation
    d_B_rho = d_b_rho;
    
    B_rho_lower = B_rho(1); B_rho_upper = B_rho(2);
    d_B_rho_lower = d_B_rho(1); d_B_rho_upper = d_B_rho(2);
    
    xi_rho = rho_e;
    B_diff_rho = B_rho_upper - B_rho_lower;
    
    theta_rho = (xi_rho - B_rho_lower) / B_diff_rho;
    
    phi_tan_rho = tan(pi * (theta_rho - 0.5));
    
    varpi_rho = (2 * pi * sec(pi * (theta_rho - 0.5))^2) / B_diff_rho;
    mu_rho = varpi_rho * (-rho_e_0 * d_iota_rho - d_B_rho_lower - ...
             (xi_rho - B_rho_lower) / B_diff_rho * (d_B_rho_upper - d_B_rho_lower));
             
    alpha_rho = (1 / varpi_rho) * (-sign(varpi_rho)*varpi_rho*gamma1_rho * phi_tan_rho - mu_rho) - S_rho;
    z_rho = d_rho_e - alpha_rho - S_rho; 

    %% ================= 4. 计算 psi 维度的控制量 =================
    N_psi = 1; if psi_e_0 < 0, N_psi = -1; end
    V_psi_0 = [1-N_psi; 1+N_psi];
    M_psi = [-1, 0.2; 0.2, 1];
    
    ups_psi = (upsilon_psi_0 - upsilon_psi_inf) * iota_psi + upsilon_psi_inf;
    d_ups_psi = (upsilon_psi_0 - upsilon_psi_inf) * d_iota_psi;
    
    b_psi = 0.5 * ups_psi * M_psi * V_psi_0 + psi_e_0 * iota_psi * [1; 1];
    d_b_psi = 0.5 * d_ups_psi * M_psi * V_psi_0 + psi_e_0 * d_iota_psi * [1; 1];
    d_kappa_psi = -k_psi_1 * kappa_psi + k_psi_2 * (chi_psi_1 + chi_psi_2);
    
    Omega_psi = [-omega_psi_1; omega_psi_2];
    B_psi = b_psi; % Ablation M4: rigid PPC, no elastic relaxation
    d_B_psi = d_b_psi;
    
    B_psi_lower = B_psi(1); B_psi_upper = B_psi(2);
    d_B_psi_lower = d_B_psi(1); d_B_psi_upper = d_B_psi(2);
    
    xi_psi = psi_e;
    B_diff_psi = B_psi_upper - B_psi_lower;
    theta_psi = (xi_psi - B_psi_lower) / B_diff_psi;
    
    
    phi_tan_psi = tan(pi * (theta_psi - 0.5));
    
    varpi_psi = (2 * pi * sec(pi * (theta_psi - 0.5))^2) / B_diff_psi;
    mu_psi = varpi_psi * (-psi_e_0 * d_iota_psi - d_B_psi_lower - ...
             (xi_psi - B_psi_lower) / B_diff_psi * (d_B_psi_upper - d_B_psi_lower));
             
    alpha_psi = (1 / varpi_psi) * (-sign(varpi_psi)*varpi_psi*gamma1_psi * phi_tan_psi - mu_psi) - S_psi;
    z_psi = d_psi_e - alpha_psi - S_psi; 
    
    % kappa_rho = 2*rho_e*sigma_rho^2/(sigma_rho^2 - rho_e^2)^2;
    % kappa_psi = 2*psi_e*sigma_psi^2/(sigma_psi^2 - psi_e^2)^2;
    
    vartheta_rho = norm(NN([alpha_rho,rho_e])) + 1;
    vartheta_psi = norm(NN([alpha_psi,psi_e])) + 1;
    
    term1=tanh(mu_rho_hat *Phi_rho^2* z_rho^2 * vartheta_rho^2 / epsilon);
    term2=tanh(mu_psi_hat *Phi_psi^2* z_psi^2 * vartheta_psi^2 / epsilon);
    
    tau_u = -(1/g) * (0.5 * K_rho * z_rho + 0.5*mu_rho_hat * vartheta_rho^2 *Phi_rho^2* z_rho * term1);
    tau_r = -(1/h) * (0.5 * K_psi * z_psi + 0.5*mu_psi_hat * vartheta_psi^2 *Phi_psi^2* z_psi * term2);
    
    dot_mu_rho_hat = -wp_rho * (-0.5 * vartheta_rho^2*Phi_rho^2*z_rho^2 + varphi_rho * mu_rho_hat);
    dot_mu_psi_hat = -wp_psi * (-0.5 * vartheta_psi^2*Phi_psi^2*z_psi^2 + varphi_psi * mu_psi_hat);
    

    tau_bu_psi = 400;tau_bu_rho = 800;
    term_rho_1 = (sign(tau_u - tau_bu_rho) + 1) * (tau_u - tau_bu_rho);
    term_rho_2 = (sign(tau_u + tau_bu_rho) - 1) * (tau_u + tau_bu_rho);
    d_chi_rho_1 = -a_rho_1 * chi_rho_1 + b_rho_1 * term_rho_1;
    d_chi_rho_2 = -a_rho_2 * chi_rho_2 + b_rho_2 * term_rho_2;
    term_psi_1 = (sign(tau_r - tau_bu_psi) + 1) * (tau_r - tau_bu_psi);
    term_psi_2 = (sign(tau_r + tau_bu_psi) - 1) * (tau_r + tau_bu_psi);
    d_chi_psi_1 = -a_psi_1 * chi_psi_1 + b_psi_1 * term_psi_1;
    d_chi_psi_2 = -a_psi_2 * chi_psi_2 + b_psi_2 * term_psi_2;
    % 模拟实际限幅函数 g(tau)
    G_psi = h;G_rho = g;
    tau_sat_psi = max(min(tau_r, tau_bu_psi), -tau_bu_psi);
    d_S_psi = -S_psi + G_psi * (tau_sat_psi - tau_r);
    % 模拟实际限幅函数 g(tau)
    tau_sat_rho = max(min(tau_u, tau_bu_rho), -tau_bu_rho); 
    d_S_rho = -S_rho + G_rho * (tau_sat_rho - tau_u);
end

 function NNv= NN(theta)
    NNv = zeros(50,1);
    for i=1:50
        paran = 0.005*i;
        param = ones(length(theta),1)*sin(0.1*i);
        NNv(i) = exp(-norm(theta-param)^2/paran);
    end
end

== matlab function abl_M4_rigidPPC/Subsystem16/Subsystem/Guidence ==
  settings: updateMethod=DISCRETE
  data: t input; x input; y input; desire input; psi input; psid output; psi_e output; rhoe output; xd output; yd output
function [psid,psi_e,rhoe,xd,yd]  = desire(t,x,y,desire,psi)
xd = desire(1);yd = desire(4);
dxd = desire(2); dyd=desire(5);
xe =x-xd;
ye =y-yd;
 rhoe = sqrt((xe)^2+(ye)^2); 
 persistent kkk2 gpsid2
% if abs(rhoe)<1
    p = atan2(10000*ye+10*dyd,10000*xe+10*dxd);
    % u1 = 0.1*dxd+10*xe;
    % u2 = 0.1*dyd+10*ye;
    % z=u1+u2*i;
    % p=angle(z);
% else
%     p = atan2(ye,xe);
% end

if isempty(kkk2)
    kkk2=0;
    gpsid2=p;
end
if p*gpsid2<-0.7*pi^2 && p>0  %Change nearly in -pi and +pi
   kkk2=kkk2-1;
end
if p*gpsid2<-0.7*pi^2 && p<0  %Change nearly in -pi and +pi
   kkk2=kkk2+1;
end
gpsid2=p;
psid=p+2*kkk2*pi;
psi_e = psi-psid;
 
 

end

== matlab function abl_M4_rigidPPC/Subsystem16/Subsystem1/MATLAB Function1 ==
  data: x1 input; dotx1 output; dotx2 output; x2 input; psid input
function [dotx1,dotx2] = desire(x1,x2,psid)
    R  = 1;
    dotx1 = x2;
    dotx2 = -2*R^2*(x1-psid)-R*x2;
end

== matlab function abl_M4_rigidPPC/Subsystem16/Subsystem1/MATLAB Function2 ==
  data: x1 input; dotx1 output; dotx2 output; x2 input; psid input
function [dotx1,dotx2] = desire(x1,x2,psid)
    R  = 1;
    dotx1 = x2;
    dotx2 = -2*R^2*(x1-psid)-R*x2;
end

== matlab function abl_M4_rigidPPC/Subsystem17/MATLAB Function8 ==
  data: x1 input; dotx1 output; dotx2 output; x2 input; dpd input
function [dotx1,dotx2] = desire(x1,x2,dpd)
    R  = 1;
    dotx1 = x2;
    dotx2 = -2*R^2*(x1-dpd)-R*x2;
end

== matlab function abl_M4_rigidPPC/Subsystem17/MATLAB Function9 ==
  data: x1 input; dotx1 output; dotx2 output; x2 input; pd input
function [dotx1,dotx2] = desire(x1,x2,pd)
    R  = 10;
    dotx1 = x2;
    dotx2 = -2*R^2*(x1-pd)-R*x2;
end

== matlab function abl_M4_rigidPPC/Subsystem18/Controler1 ==
  settings: updateMethod=DISCRETE
  data: t input; psi_d input; dpsid input; ddpsid input; psi_e input; rho_e input; tau_sat_rho output; tau_sat_psi output; alpha_psi output; alpha_rho output; B_psi output; B_rho output; z_rho output; desire input; u input; v input; r input; mu_rho_hat input; mu_psi_hat input; kappa_rho input; kappa_psi input; dot_mu_rho_hat output; dot_mu_psi_hat output; d_kappa_rho output; d_kappa_psi output; d_chi_rho_1 output; d_chi_rho_2 output; d_chi_psi_1 output; d_chi_psi_2 output; chi_rho_1 input; chi_rho_2 input; chi_psi_1 input; chi_psi_2 input; S_rho input; S_psi input; d_S_rho output; d_S_psi output
% function [tau_u,tau_r,alpha_psi,alpha_rho,dot_mu_rho_hat,dot_mu_psi_hat,sigma_rho,sigma_psi,z_rho,z_psi,term1 ,dpsie] = controller(t,psi_d,dpsid,ddpsid,psi_e, rho_e,desire,u, v, r,mu_rho_hat,mu_psi_hat)
% dxd = desire(2);ddxd = desire(3);dyd = desire(5);ddyd = desire(6);
% dpsie = r-dpsid;
% drhoe = u*cos(psi_e)+v*sin(psi_e)-dxd*cos(psi_d)-dyd*sin(psi_d);

% % epsilon = 0.05;

% % varkappa_rho =0.001;varkappa_psi=0.0005;
% % varpi_rho =2;varpi_psi =10;
% % k_rho=1.5;k_psi=10;
% % if rho_e<0.07
% %    varpi_rho =20;
% % end
% % if psi_e<0.1
% %    varpi_psi =50;
% % end
% % Tc_rho =16;Tc_psi =5;alpha=0.8;
% % sigma_rho0 =5;sigma_psi0 =2;
% % sigma_rho_inf =0.2;sigma_psi_inf=0.05;
% % Phi_rho=6*7;Phi_psi=8*7;
% 
% m11=25.8;m33=2.76;
% epsilon = 0.05;

% varkappa_rho =0.01;varkappa_psi=0.08;
% varpi_rho =1;varpi_psi =0.001;
% k_rho=100;k_psi=10;
% % if rho_e<0.07
% %    varpi_rho =20;
% % end
% % if psi_e<0.1
% %    varpi_psi =50;
% % end
% Tc_rho =25;Tc_psi =6;alpha=0.8;
% sigma_rho0 =20;sigma_psi0 =3;
% sigma_rho_inf =0.5;sigma_psi_inf=0.2;
% Phi_rho=0.01;Phi_psi=1;
% 

% 
% if t < Tc_rho
%      q_rho = 1-sin(pi*t/(2*Tc_rho));
%      dq_rho = -cos(pi*t/(2*Tc_rho))*pi/(2*Tc_rho);
% else
%     q_rho=0;
%     dq_rho=0;
% end
% if t < Tc_psi
%      q_psi = 1-sin(pi*t/(2*Tc_psi));
%      dq_psi = -cos(pi*t/(2*Tc_psi))*pi/(2*Tc_psi);
% else
%     q_psi = 0;
%     dq_psi=0;
% end
% 
% sigma_rho = (sigma_rho0 - sigma_rho_inf) * q_rho + sigma_rho_inf;
% sigma_psi = (sigma_psi0 - sigma_psi_inf) * q_psi + sigma_psi_inf;
% dsigma_rho = (sigma_rho0 - sigma_rho_inf)*dq_rho;
% dsigma_psi = (sigma_psi0 - sigma_psi_inf)*dq_psi;
% 
% alpha_rho =(1/sigma_rho^2)*(rho_e*sigma_rho*dsigma_rho-0.5*k_rho*(sigma_rho^2-rho_e^2)*rho_e-0*rho_e);
% alpha_psi =(1/sigma_psi^2)*(psi_e*sigma_psi*dsigma_psi-0.5*k_psi*(sigma_psi^2-psi_e^2)*psi_e);




function [tau_sat_rho,tau_sat_psi,alpha_psi, alpha_rho,B_psi,B_rho, z_rho, dot_mu_rho_hat, dot_mu_psi_hat, d_kappa_rho, d_kappa_psi,d_chi_rho_1,d_chi_rho_2,d_chi_psi_1,d_chi_psi_2,d_S_rho,d_S_psi] = LowLevel_Controller(t, psi_d,dpsid,ddpsid,psi_e, rho_e,desire,u, v, r,mu_rho_hat,mu_psi_hat,kappa_rho, kappa_psi,chi_rho_1,chi_rho_2,chi_psi_1,chi_psi_2,S_rho,S_psi)
    dxd = desire(2);ddxd = desire(3);dyd = desire(5);ddyd = desire(6);
    d_psi_e = r-dpsid;
    d_rho_e = u*cos(psi_e)-v*sin(psi_e)-dxd*cos(psi_d)-dyd*sin(psi_d); 
   % 移动目标围捕底层控制：预设时间与预设精度障碍李雅普诺夫控制器
    %
    % id: 当前智能体编号
    % A_raw: 全局通信拓扑矩阵 (NxN)
    
   %% ================= 0. 拓扑切换自动重启与初值捕获机制 =================
    persistent rho_e_0 psi_e_0;
    
    % 初始化阶段 (t = 0)
    if isempty(rho_e_0)
        rho_e_0 = rho_e;
        psi_e_0 = psi_e;
    end
   
    
    % Tracking PPC keeps the original time base; topology restart is handled in observer/guidance.
    t_local = t;

    %% ================= 1. 控制器参数配置 =================
    %Tc = 10.0; % 预设收敛时间 T_c
    
    % --- 径向误差(rho)参数 ---
    upsilon_rho_0 = 10;     
    upsilon_rho_inf = 0.2;          
    omega_rho_1 = 5.5; omega_rho_2 = 5.5;       
    gamma1_rho = 0.35;        
    k_rho_1 = 1.0;           
    k_rho_2 = 1.0;              
    Phi_rho=1;Phi_psi=2;
    K_psi = 135;K_rho = 0.018;
    m11=24.9;m33=2.86;
    h= 1/m33;
    g = cos(psi_e)/m11;

    % --- 航向误差(psi)参数 ---
    upsilon_psi_0 = 2*pi/5; 
    upsilon_psi_inf = 0.02;
    omega_psi_1 = 1; omega_psi_2 = 1;
    gamma1_psi = 4.0;
    k_psi_1 = 1.0;
    k_psi_2 = 1.0;  
    epsilon = 0.03;

    a_rho_1 = 300;a_rho_2 = 1000;b_rho_1 = 1;b_rho_2 = 1;
    a_psi_1 = 1000;a_psi_2 = 1000;b_psi_1 = 1;b_psi_2 = 1;
    wp_rho =0.001;wp_psi=0.001;
    varphi_rho =2;varphi_psi =1;
    %% ================= 2. 预设时间收敛函数 (使用 t_local 重启) =================
    % 严格对应公式 (0.4)
    Tc_psi = 2;
    if t_local < Tc_psi
        iota_psi = 1 - sin(pi * t_local / (2 * Tc_psi));
        d_iota_psi = -(pi / (2 * Tc_psi)) * cos(pi * t_local / (2 * Tc_psi));
    else
        iota_psi = 0;
        d_iota_psi = 0;
    end

    Tc_rho = 10;
    if t_local < Tc_rho
        iota_rho = 1 - sin(pi * t_local / (2 * Tc_rho));
        d_iota_rho = -(pi / (2 * Tc_rho)) * cos(pi * t_local / (2 * Tc_rho));
    else
        iota_rho = 0;
        d_iota_rho = 0;
    end

    %% ================= 3. 计算 rho 维度的控制量 =================
    N_rho = 1; if rho_e_0 < 0, N_rho = -1; end
    V_rho_0 = [1- N_rho; 1+N_rho];
    M_rho = [-1, -0.2; 0.2, 1];
    
    ups_rho = (upsilon_rho_0 - upsilon_rho_inf) * iota_rho + upsilon_rho_inf;
    d_ups_rho = (upsilon_rho_0 - upsilon_rho_inf) * d_iota_rho;
    
    b_rho = 0.5 * ups_rho * M_rho * V_rho_0 + rho_e_0 * iota_rho * [1; 1];
    d_b_rho = 0.5 * d_ups_rho * M_rho * V_rho_0 + rho_e_0 * d_iota_rho * [1; 1];
    d_kappa_rho = -k_rho_1 * kappa_rho + k_rho_2 * (chi_rho_1 + chi_rho_2);
    
    Omega_rho = [-omega_rho_1; omega_rho_2];
    B_rho = b_rho; % Ablation M4: rigid PPC, no elastic relaxation
    d_B_rho = d_b_rho;
    
    B_rho_lower = B_rho(1); B_rho_upper = B_rho(2);
    d_B_rho_lower = d_B_rho(1); d_B_rho_upper = d_B_rho(2);
    
    xi_rho = rho_e;
    B_diff_rho = B_rho_upper - B_rho_lower;
    
    theta_rho = (xi_rho - B_rho_lower) / B_diff_rho;
    
    phi_tan_rho = tan(pi * (theta_rho - 0.5));
    
    varpi_rho = (2 * pi * sec(pi * (theta_rho - 0.5))^2) / B_diff_rho;
    mu_rho = varpi_rho * (-rho_e_0 * d_iota_rho - d_B_rho_lower - ...
             (xi_rho - B_rho_lower) / B_diff_rho * (d_B_rho_upper - d_B_rho_lower));
             
    alpha_rho = (1 / varpi_rho) * (-sign(varpi_rho)*varpi_rho*gamma1_rho * phi_tan_rho - mu_rho) - S_rho;
    z_rho = d_rho_e - alpha_rho - S_rho; 

    %% ================= 4. 计算 psi 维度的控制量 =================
    N_psi = 1; if psi_e_0 < 0, N_psi = -1; end
    V_psi_0 = [1-N_psi; 1+N_psi];
    M_psi = [-1, 0.2; 0.2, 1];
    
    ups_psi = (upsilon_psi_0 - upsilon_psi_inf) * iota_psi + upsilon_psi_inf;
    d_ups_psi = (upsilon_psi_0 - upsilon_psi_inf) * d_iota_psi;
    
    b_psi = 0.5 * ups_psi * M_psi * V_psi_0 + psi_e_0 * iota_psi * [1; 1];
    d_b_psi = 0.5 * d_ups_psi * M_psi * V_psi_0 + psi_e_0 * d_iota_psi * [1; 1];
    d_kappa_psi = -k_psi_1 * kappa_psi + k_psi_2 * (chi_psi_1 + chi_psi_2);
    
    Omega_psi = [-omega_psi_1; omega_psi_2];
    B_psi = b_psi; % Ablation M4: rigid PPC, no elastic relaxation
    d_B_psi = d_b_psi;
    
    B_psi_lower = B_psi(1); B_psi_upper = B_psi(2);
    d_B_psi_lower = d_B_psi(1); d_B_psi_upper = d_B_psi(2);
    
    xi_psi = psi_e;
    B_diff_psi = B_psi_upper - B_psi_lower;
    theta_psi = (xi_psi - B_psi_lower) / B_diff_psi;
    
    
    phi_tan_psi = tan(pi * (theta_psi - 0.5));
    
    varpi_psi = (2 * pi * sec(pi * (theta_psi - 0.5))^2) / B_diff_psi;
    mu_psi = varpi_psi * (-psi_e_0 * d_iota_psi - d_B_psi_lower - ...
             (xi_psi - B_psi_lower) / B_diff_psi * (d_B_psi_upper - d_B_psi_lower));
             
    alpha_psi = (1 / varpi_psi) * (-sign(varpi_psi)*varpi_psi*gamma1_psi * phi_tan_psi - mu_psi) - S_psi;
    z_psi = d_psi_e - alpha_psi - S_psi; 
    
    % kappa_rho = 2*rho_e*sigma_rho^2/(sigma_rho^2 - rho_e^2)^2;
    % kappa_psi = 2*psi_e*sigma_psi^2/(sigma_psi^2 - psi_e^2)^2;
    
    vartheta_rho = norm(NN([alpha_rho,rho_e])) + 1;
    vartheta_psi = norm(NN([alpha_psi,psi_e])) + 1;
    
    term1=tanh(mu_rho_hat *Phi_rho^2* z_rho^2 * vartheta_rho^2 / epsilon);
    term2=tanh(mu_psi_hat *Phi_psi^2* z_psi^2 * vartheta_psi^2 / epsilon);
    
    tau_u = -(1/g) * (0.5 * K_rho * z_rho + 0.5*mu_rho_hat * vartheta_rho^2 *Phi_rho^2* z_rho * term1);
    tau_r = -(1/h) * (0.5 * K_psi * z_psi + 0.5*mu_psi_hat * vartheta_psi^2 *Phi_psi^2* z_psi * term2);
    
    dot_mu_rho_hat = -wp_rho * (-0.5 * vartheta_rho^2*Phi_rho^2*z_rho^2 + varphi_rho * mu_rho_hat);
    dot_mu_psi_hat = -wp_psi * (-0.5 * vartheta_psi^2*Phi_psi^2*z_psi^2 + varphi_psi * mu_psi_hat);
    

    tau_bu_psi = 400;tau_bu_rho = 800;
    term_rho_1 = (sign(tau_u - tau_bu_rho) + 1) * (tau_u - tau_bu_rho);
    term_rho_2 = (sign(tau_u + tau_bu_rho) - 1) * (tau_u + tau_bu_rho);
    d_chi_rho_1 = -a_rho_1 * chi_rho_1 + b_rho_1 * term_rho_1;
    d_chi_rho_2 = -a_rho_2 * chi_rho_2 + b_rho_2 * term_rho_2;
    term_psi_1 = (sign(tau_r - tau_bu_psi) + 1) * (tau_r - tau_bu_psi);
    term_psi_2 = (sign(tau_r + tau_bu_psi) - 1) * (tau_r + tau_bu_psi);
    d_chi_psi_1 = -a_psi_1 * chi_psi_1 + b_psi_1 * term_psi_1;
    d_chi_psi_2 = -a_psi_2 * chi_psi_2 + b_psi_2 * term_psi_2;
    % 模拟实际限幅函数 g(tau)
    G_psi = h;G_rho = g;
    tau_sat_psi = max(min(tau_r, tau_bu_psi), -tau_bu_psi);
    d_S_psi = -S_psi + G_psi * (tau_sat_psi - tau_r);
    % 模拟实际限幅函数 g(tau)
    tau_sat_rho = max(min(tau_u, tau_bu_rho), -tau_bu_rho); 
    d_S_rho = -S_rho + G_rho * (tau_sat_rho - tau_u);
end

 function NNv= NN(theta)
    NNv = zeros(50,1);
    for i=1:50
        paran = 0.005*i;
        param = ones(length(theta),1)*sin(0.1*i);
        NNv(i) = exp(-norm(theta-param)^2/paran);
    end
end

== matlab function abl_M4_rigidPPC/MATLAB Function1 ==
  settings: updateMethod=DISCRETE
  data: t input; dp_hat_i output; p0 input; v0 input; p_hat_all input; v_hat_all input; p_d_all input; id input; A_row input; beta input; p_offset input; dv_hat_i output; dp_d_i output
function [dp_hat_i, dv_hat_i, dp_d_i] = Follower_Model(t, p0, v0, p_hat_all, v_hat_all, p_d_all, id, A_row, beta, p_offset)
    % 输入说明:
    % t: 仿真时间 (Clock)
    % p0, v0: 领航者真实状态 (仅在beta_i > 0时起作用)
    % p_hat_all, v_hat_all, p_d_all: 所有跟随者的状态矩阵 (外部合并后传入)
    % id: 当前智能体编号
    % A_row: 当前智能体对其他人的邻接权重 (用于检测网络拓扑变化)
    % beta_i: 当前智能体是否能直接观测到领航者 (1或0)
    % p_offset: 期望与目标的相对编队位置偏置 (2x1 向量)

    % --- 仿真参数设定 ---
    kp_l = 0.5; 
    phi_p = 2.0; 
    Ta = 5.0;         % 规定观测器收敛时间
    Omega_bar = 4; 
    k1 = 0.1; 
    lambda = 1.0; 
    Tp = 10.0;      % 规定围住控制形成的时间
    d_avoid = 10;    % 避碰距离 d
    mu = 20;         % 避碰范围上限 mu

    % === 自动重启机制核心逻辑 ===
    % 使用 persistent 变量存储上一时刻的拓扑和最近一次的切换时间 tk
    persistent tk A_row_prev;
    
    if isempty(tk)
        tk = 0;
        A_row_prev = A_row;
    end
    
    % 检测到邻接权重矩阵发生改变，说明有智能体加入/退出，更新重启时刻 tk
    if any(A_row ~= A_row_prev)
        tk = t;
        A_row_prev = A_row;
    end
    
    % 计算自上次拓扑切换以来经过的“局部时间”
    t_local = t - tk; 
    % ===========================

    p_hat_i = p_hat_all(2*(id-1)+1:2*id);
    v_hat_i = v_hat_all(2*(id-1)+1:2*id);
    p_d_i = p_d_all(2*(id-1)+1:2*id);

    %% ---------------- A. 移动目标规定时间观测器 ----------------
    sum_p = zeros(size(p_hat_i));
    sum_v = zeros(size(v_hat_i));
    % 这里的循环处理完美契合“无标签”特性：不管是谁，只要 A_row(j)>0 就计算
    for j = 1:size(beta, 1)
        if A_row(id,j) > 0 && j ~= id
            sum_p = sum_p + A_row(id,j) * (p_hat_i - p_hat_all(2*(j-1)+1:2*j));
            sum_v = sum_v + A_row(id,j) * (v_hat_i - v_hat_all(2*(j-1)+1:2*j));
        end
    end
    
    eta_ip = sum_p + beta(id) * (p_hat_i - p0);
    eta_iv = sum_v + beta(id) * (v_hat_i - v0);

    % 观测器时变增益 kp (基于局部时间 t_local 重启)
    % 引入 -0.01 防止时间刚好等于 Ta 时分母为 0
    if t_local < Ta - 0.001 
        kp = kp_l + 1/(2*phi_p) + 2/(Ta - t_local);
    else
        kp = kp_l + 1/(2*phi_p);
    end

    sig_eta_iv = sign(eta_iv); 
    dp_hat_i = v_hat_i - kp * eta_ip;
    dv_hat_i = -kp * eta_iv - Omega_bar * sig_eta_iv;

    %% ---------------- B. 无标签目标围捕导航层 ----------------
    % 导航层时变增益 k (基于局部时间 t_local 重启)
    if t_local < Tp - 0.2
        k_gain = k1 + 0.01 + lambda/(Tp - t_local);
    else
        k_gain = k1 + 0.01;
    end

    p_tilde_d_i = p_d_i - p_hat_i - 0*p_offset(:,id); 
    m_gain = 100;
    sum_avoid = zeros(size(p_d_i));
    for j = 1:size(beta, 1)
        if A_row(id,j) > 0 && j ~= id
            p_d_ij = p_d_i - p_d_all(2*(j-1)+1:2*j);
            norm_p = norm(p_d_ij);
            
            if norm_p > d_avoid && norm_p <= mu
                alpha_val = 1/(norm_p - d_avoid) - 1/(mu - d_avoid);
            else
                alpha_val = 0; % 超出感知范围，或者发生了不可逆穿透，斥力置0防崩溃
            end
            
            if norm_p > 0
                % + 号表示顺着 p_d_ij 的方向把自己推开
                sum_avoid = sum_avoid + m_gain * alpha_val * (p_d_ij / norm_p);
            end
        end
    end
    p_d_ij = p_d_i - p_hat_i;
    norm_p = norm(p_d_ij);
            
    if norm_p > d_avoid && norm_p <= mu
        alpha_val = 1/(norm_p - d_avoid) - 1/(mu - d_avoid);
    else
        alpha_val = 0; % 超出感知范围，或者发生了不可逆穿透，斥力置0防崩溃
    end
    
    if norm_p > 0
        % + 号表示顺着 p_d_ij 的方向把自己推开
        sum_avoid = sum_avoid + m_gain * alpha_val * (p_d_ij / norm_p);
    end
    % v_d_i = 速度前馈 - 引力 + 斥力
    v_d_i = v_hat_i - k_gain *(p_tilde_d_i -sum_avoid);
    dp_d_i = v_d_i;
end
